simulink model "rpoco16"  (R2013a)
settings: Solver=VariableStepDiscrete  SolverMode=SingleTasking  StartTime=0.0  StopTime=10.0  RelTol=1e-3
libraries: xbsIndex_r4 x7152, casper_library_misc x156, casper_library_multipliers x68, casper_library_sources x8, xps_library x5, casper_library_delays x1
(part 3 of 84)

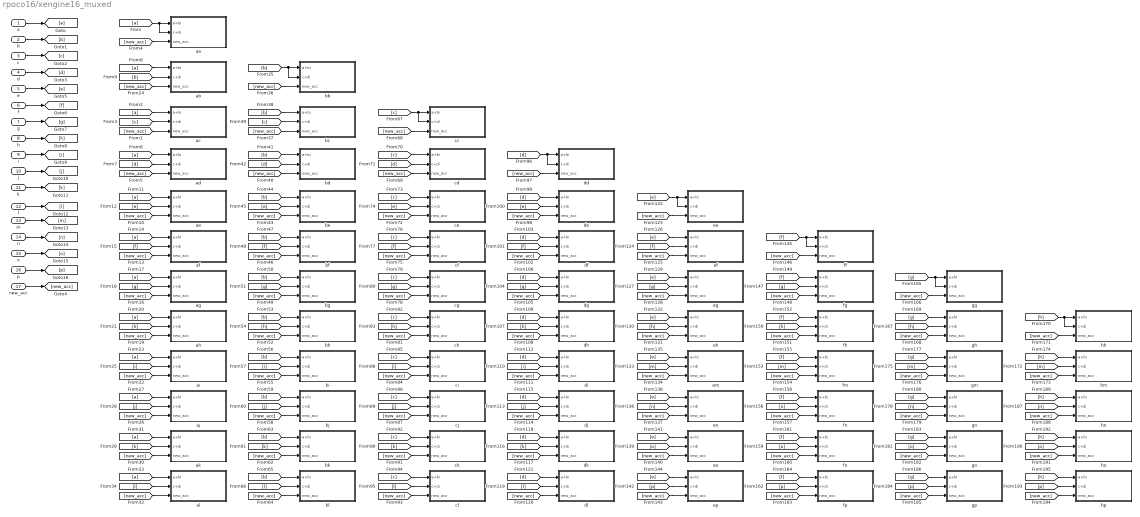
== system rpoco16/xengine16_muxed ==
  a : Inport
  b : Inport  Port=2
  c : Inport  Port=3
  d : Inport  Port=4
  e : Inport  Port=5
  f : Inport  Port=6
  g : Inport  Port=7
  h : Inport  Port=8
  i : Inport  Port=9
  j : Inport  Port=10
  k : Inport  Port=11
  l : Inport  Port=12
  m : Inport  Port=13
  n : Inport  Port=14
  o : Inport  Port=15
  p : Inport  Port=16
  new_acc : Inport  Port=17
  aa : Subsystem
  ab : Subsystem
  ac : Subsystem
  ad : Subsystem
  ae : Subsystem
  af : Subsystem
  ag : Subsystem
  ah : Subsystem
  ai : Subsystem
  aj : Subsystem
  ak : Subsystem
  al : Subsystem
  bb : Subsystem
  bc : Subsystem
  bd : Subsystem
  be : Subsystem
  bf : Subsystem
  bg : Subsystem
  bh : Subsystem
  bi : Subsystem
  bj : Subsystem
  bk : Subsystem
  bl : Subsystem
  cc : Subsystem
  cd : Subsystem
  ce : Subsystem
  cf : Subsystem
  cg : Subsystem
  ch : Subsystem
  ci : Subsystem
  cj : Subsystem
  ck : Subsystem
  cl : Subsystem
  dd : Subsystem
  de : Subsystem
  df : Subsystem
  dg : Subsystem
  dh : Subsystem
  di : Subsystem
  dj : Subsystem
  dk : Subsystem
  dl : Subsystem
  ee : Subsystem
  ef : Subsystem
  eg : Subsystem
  eh : Subsystem
  em : Subsystem
  en : Subsystem
  eo : Subsystem
  ep : Subsystem
  ff : Subsystem
  fg : Subsystem
  fh : Subsystem
  fm : Subsystem
  fn : Subsystem
  fo : Subsystem
  fp : Subsystem
  gg : Subsystem
  gh : Subsystem
  gm : Subsystem
  gn : Subsystem
  go : Subsystem
  gp : Subsystem
  hh : Subsystem
  hm : Subsystem
  hn : Subsystem
  ho : Subsystem
  hp : Subsystem
  wires:
  a/1 -> [a]
  b/1 -> [b]
  c/1 -> [c]
  d/1 -> [d]
  new_acc/1 -> [new_acc]
  [a] -> aa/2(c+di), aa/1(a+bi)
  [new_acc] -> aa/3(new_acc)
  e/1 -> [e]
  f/1 -> [f]
  g/1 -> [g]
  h/1 -> [h]
  [new_acc] -> ab/3(new_acc)
  [a] -> ab/1(a+bi)
  [b] -> ab/2(c+di)
  p/1 -> [p]
  o/1 -> [o]
  n/1 -> [n]
  m/1 -> [m]
  l/1 -> [l]
  k/1 -> [k]
  j/1 -> [j]
  i/1 -> [i]
  [new_acc] -> ac/3(new_acc)
  [a] -> ac/1(a+bi)
  [c] -> ac/2(c+di)
  [new_acc] -> ad/3(new_acc)
  [a] -> ad/1(a+bi)
  [d] -> ad/2(c+di)
  [new_acc] -> ae/3(new_acc)
  [a] -> ae/1(a+bi)
  [e] -> ae/2(c+di)
  [new_acc] -> af/3(new_acc)
  [a] -> af/1(a+bi)
  [f] -> af/2(c+di)
  [new_acc] -> ag/3(new_acc)
  [a] -> ag/1(a+bi)
  [g] -> ag/2(c+di)
  [new_acc] -> ah/3(new_acc)
  [a] -> ah/1(a+bi)
  [h] -> ah/2(c+di)
  [new_acc] -> ai/3(new_acc)
  [a] -> ai/1(a+bi)
  [i] -> ai/2(c+di)
  [new_acc] -> aj/3(new_acc)
  [a] -> aj/1(a+bi)
  [j] -> aj/2(c+di)
  [new_acc] -> al/3(new_acc)
  [a] -> al/1(a+bi)
  [l] -> al/2(c+di)
  [b] -> bb/1(a+bi), bb/2(c+di)
  [new_acc] -> bb/3(new_acc)
  [new_acc] -> bc/3(new_acc)
  [b] -> bc/1(a+bi)
  [c] -> bc/2(c+di)
  [new_acc] -> bd/3(new_acc)
  [b] -> bd/1(a+bi)
  [d] -> bd/2(c+di)
  [new_acc] -> be/3(new_acc)
  [b] -> be/1(a+bi)
  [e] -> be/2(c+di)
  [new_acc] -> bf/3(new_acc)
  [b] -> bf/1(a+bi)
  [f] -> bf/2(c+di)
  [new_acc] -> bg/3(new_acc)
  [b] -> bg/1(a+bi)
  [g] -> bg/2(c+di)
  [new_acc] -> bh/3(new_acc)
  [b] -> bh/1(a+bi)
  [h] -> bh/2(c+di)
  [new_acc] -> bi/3(new_acc)
  [b] -> bi/1(a+bi)
  [i] -> bi/2(c+di)
  [new_acc] -> bj/3(new_acc)
  [b] -> bj/1(a+bi)
  [j] -> bj/2(c+di)
  [new_acc] -> bl/3(new_acc)
  [b] -> bl/1(a+bi)
  [l] -> bl/2(c+di)
  [c] -> cc/2(c+di), cc/1(a+bi)
  [new_acc] -> cc/3(new_acc)
  [new_acc] -> cd/3(new_acc)
  [c] -> cd/1(a+bi)
  [d] -> cd/2(c+di)
  [new_acc] -> ce/3(new_acc)
  [c] -> ce/1(a+bi)
  [e] -> ce/2(c+di)
  [new_acc] -> cf/3(new_acc)
  [c] -> cf/1(a+bi)
  [f] -> cf/2(c+di)
  [new_acc] -> cg/3(new_acc)
  [c] -> cg/1(a+bi)
  [g] -> cg/2(c+di)
  [new_acc] -> ch/3(new_acc)
  [c] -> ch/1(a+bi)
  [h] -> ch/2(c+di)
  [new_acc] -> ci/3(new_acc)
  [c] -> ci/1(a+bi)
  [i] -> ci/2(c+di)
  [new_acc] -> cj/3(new_acc)
  [c] -> cj/1(a+bi)
  [j] -> cj/2(c+di)
  [new_acc] -> cl/3(new_acc)
  [c] -> cl/1(a+bi)
  [l] -> cl/2(c+di)
  [d] -> dd/1(a+bi), dd/2(c+di)
  [new_acc] -> dd/3(new_acc)
  [new_acc] -> de/3(new_acc)
  [d] -> de/1(a+bi)
  [e] -> de/2(c+di)
  [new_acc] -> df/3(new_acc)
  [d] -> df/1(a+bi)
  [f] -> df/2(c+di)
  [new_acc] -> dg/3(new_acc)
  [d] -> dg/1(a+bi)
  [g] -> dg/2(c+di)
  [new_acc] -> dh/3(new_acc)
  [d] -> dh/1(a+bi)
  [h] -> dh/2(c+di)
  [new_acc] -> di/3(new_acc)
  [d] -> di/1(a+bi)
  [i] -> di/2(c+di)
  [new_acc] -> dj/3(new_acc)
  [d] -> dj/1(a+bi)
  [j] -> dj/2(c+di)
  [new_acc] -> dl/3(new_acc)
  [d] -> dl/1(a+bi)
  [l] -> dl/2(c+di)
  [e] -> ee/2(c+di), ee/1(a+bi)
  [new_acc] -> ee/3(new_acc)
  [new_acc] -> ef/3(new_acc)
  [e] -> ef/1(a+bi)
  [f] -> ef/2(c+di)
  [new_acc] -> eg/3(new_acc)
  [e] -> eg/1(a+bi)
  [g] -> eg/2(c+di)
  [new_acc] -> eh/3(new_acc)
  [e] -> eh/1(a+bi)
  [h] -> eh/2(c+di)
  [new_acc] -> em/3(new_acc)
  [e] -> em/1(a+bi)
  [m] -> em/2(c+di)
  [new_acc] -> en/3(new_acc)
  [e] -> en/1(a+bi)
  [n] -> en/2(c+di)
  [new_acc] -> eo/3(new_acc)
  [e] -> eo/1(a+bi)
  [o] -> eo/2(c+di)
  [new_acc] -> ep/3(new_acc)
  [e] -> ep/1(a+bi)
  [p] -> ep/2(c+di)
  [f] -> ff/1(a+bi), ff/2(c+di)
  [new_acc] -> fg/3(new_acc)
  [f] -> fg/1(a+bi)
  [g] -> fg/2(c+di)
  [new_acc] -> ff/3(new_acc)
  [new_acc] -> fh/3(new_acc)
  [f] -> fh/1(a+bi)
  [h] -> fh/2(c+di)
  [new_acc] -> fm/3(new_acc)
  [f] -> fm/1(a+bi)
  [m] -> fm/2(c+di)
  [new_acc] -> fn/3(new_acc)
  [f] -> fn/1(a+bi)
  [n] -> fn/2(c+di)
  [new_acc] -> fo/3(new_acc)
  [f] -> fo/1(a+bi)
  [o] -> fo/2(c+di)
  [new_acc] -> fp/3(new_acc)
  [f] -> fp/1(a+bi)
  [p] -> fp/2(c+di)
  [g] -> gg/2(c+di), gg/1(a+bi)
  [new_acc] -> gg/3(new_acc)
  [new_acc] -> gh/3(new_acc)
  [g] -> gh/1(a+bi)
  [h] -> gh/2(c+di)
  [h] -> hh/1(a+bi), hh/2(c+di)
  [new_acc] -> hh/3(new_acc)
  [new_acc] -> hm/3(new_acc)
  [h] -> hm/1(a+bi)
  [m] -> hm/2(c+di)
  [new_acc] -> gm/3(new_acc)
  [g] -> gm/1(a+bi)
  [m] -> gm/2(c+di)
  [new_acc] -> gn/3(new_acc)
  [g] -> gn/1(a+bi)
  [n] -> gn/2(c+di)
  [new_acc] -> go/3(new_acc)
  [g] -> go/1(a+bi)
  [o] -> go/2(c+di)
  [new_acc] -> gp/3(new_acc)
  [g] -> gp/1(a+bi)
  [p] -> gp/2(c+di)
  [new_acc] -> hn/3(new_acc)
  [h] -> hn/1(a+bi)
  [n] -> hn/2(c+di)
  [new_acc] -> ho/3(new_acc)
  [h] -> ho/1(a+bi)
  [o] -> ho/2(c+di)
  [new_acc] -> hp/3(new_acc)
  [h] -> hp/1(a+bi)
  [p] -> hp/2(c+di)
  [new_acc] -> ak/3(new_acc)
  [a] -> ak/1(a+bi)
  [k] -> ak/2(c+di)
  [new_acc] -> bk/3(new_acc)
  [b] -> bk/1(a+bi)
  [k] -> bk/2(c+di)
  [new_acc] -> ck/3(new_acc)
  [c] -> ck/1(a+bi)
  [k] -> ck/2(c+di)
  [new_acc] -> dk/3(new_acc)
  [d] -> dk/1(a+bi)
  [k] -> dk/2(c+di)

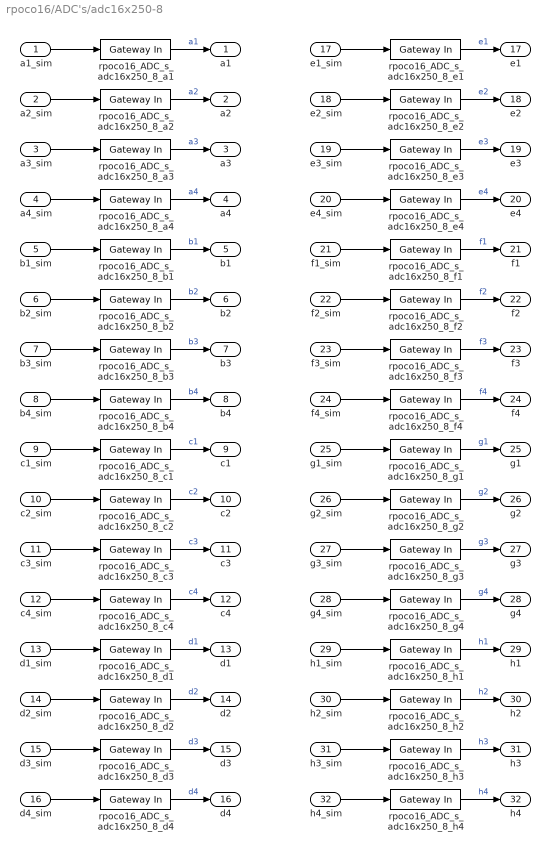
== system rpoco16/ADC's/adc16x250-8 ==
  a1_sim : Inport
  a2_sim : Inport  Port=2
  a3_sim : Inport  Port=3
  a4_sim : Inport  Port=4
  b1_sim : Inport  Port=5
  b2_sim : Inport  Port=6
  b3_sim : Inport  Port=7
  b4_sim : Inport  Port=8
  c1_sim : Inport  Port=9
  c2_sim : Inport  Port=10
  c3_sim : Inport  Port=11
  c4_sim : Inport  Port=12
  d1_sim : Inport  Port=13
  d2_sim : Inport  Port=14
  d3_sim : Inport  Port=15
  d4_sim : Inport  Port=16
  e1_sim : Inport  Port=17
  e2_sim : Inport  Port=18
  e3_sim : Inport  Port=19
  e4_sim : Inport  Port=20
  f1_sim : Inport  Port=21
  f2_sim : Inport  Port=22
  f3_sim : Inport  Port=23
  f4_sim : Inport  Port=24
  g1_sim : Inport  Port=25
  g2_sim : Inport  Port=26
  g3_sim : Inport  Port=27
  g4_sim : Inport  Port=28
  h1_sim : Inport  Port=29
  h2_sim : Inport  Port=30
  h3_sim : Inport  Port=31
  h4_sim : Inport  Port=32
  rpoco16_ADC_s_adc16x250_8_a{1..4} (4 alike) : xbsIndex_r4/Gateway In  gui_display_data_type=Fixed-point  arith_type="Signed  (2's comp)"  n_bits=8  bin_pt=7  preci_type=Single  exp_width=8  frac_width=24  quantization="Round  (unbiased: +/- Inf)"  overflow=Saturate  period=1  dbl_ovrd=off  timing_constraint=None  locs_specified=off  LOCs={}  UseAsADC=off  ADCChannel='1'  inherit_from_input=off  hdl_port=on  block_type=gatewayin
  rpoco16_ADC_s_adc16x250_8_b{1..4} (4 alike) : xbsIndex_r4/Gateway In  gui_display_data_type=Fixed-point  arith_type="Signed  (2's comp)"  n_bits=8  bin_pt=7  preci_type=Single  exp_width=8  frac_width=24  quantization="Round  (unbiased: +/- Inf)"  overflow=Saturate  period=1  dbl_ovrd=off  timing_constraint=None  locs_specified=off  LOCs={}  UseAsADC=off  ADCChannel='1'  inherit_from_input=off  hdl_port=on  block_type=gatewayin
  rpoco16_ADC_s_adc16x250_8_c{1..4} (4 alike) : xbsIndex_r4/Gateway In  gui_display_data_type=Fixed-point  arith_type="Signed  (2's comp)"  n_bits=8  bin_pt=7  preci_type=Single  exp_width=8  frac_width=24  quantization="Round  (unbiased: +/- Inf)"  overflow=Saturate  period=1  dbl_ovrd=off  timing_constraint=None  locs_specified=off  LOCs={}  UseAsADC=off  ADCChannel='1'  inherit_from_input=off  hdl_port=on  block_type=gatewayin
  rpoco16_ADC_s_adc16x250_8_d{1..4} (4 alike) : xbsIndex_r4/Gateway In  gui_display_data_type=Fixed-point  arith_type="Signed  (2's comp)"  n_bits=8  bin_pt=7  preci_type=Single  exp_width=8  frac_width=24  quantization="Round  (unbiased: +/- Inf)"  overflow=Saturate  period=1  dbl_ovrd=off  timing_constraint=None  locs_specified=off  LOCs={}  UseAsADC=off  ADCChannel='1'  inherit_from_input=off  hdl_port=on  block_type=gatewayin
  rpoco16_ADC_s_adc16x250_8_e{1..4} (4 alike) : xbsIndex_r4/Gateway In  gui_display_data_type=Fixed-point  arith_type="Signed  (2's comp)"  n_bits=8  bin_pt=7  preci_type=Single  exp_width=8  frac_width=24  quantization="Round  (unbiased: +/- Inf)"  overflow=Saturate  period=1  dbl_ovrd=off  timing_constraint=None  locs_specified=off  LOCs={}  UseAsADC=off  ADCChannel='1'  inherit_from_input=off  hdl_port=on  block_type=gatewayin
  rpoco16_ADC_s_adc16x250_8_f{1..4} (4 alike) : xbsIndex_r4/Gateway In  gui_display_data_type=Fixed-point  arith_type="Signed  (2's comp)"  n_bits=8  bin_pt=7  preci_type=Single  exp_width=8  frac_width=24  quantization="Round  (unbiased: +/- Inf)"  overflow=Saturate  period=1  dbl_ovrd=off  timing_constraint=None  locs_specified=off  LOCs={}  UseAsADC=off  ADCChannel='1'  inherit_from_input=off  hdl_port=on  block_type=gatewayin
  rpoco16_ADC_s_adc16x250_8_g{1..4} (4 alike) : xbsIndex_r4/Gateway In  gui_display_data_type=Fixed-point  arith_type="Signed  (2's comp)"  n_bits=8  bin_pt=7  preci_type=Single  exp_width=8  frac_width=24  quantization="Round  (unbiased: +/- Inf)"  overflow=Saturate  period=1  dbl_ovrd=off  timing_constraint=None  locs_specified=off  LOCs={}  UseAsADC=off  ADCChannel='1'  inherit_from_input=off  hdl_port=on  block_type=gatewayin
  rpoco16_ADC_s_adc16x250_8_h{1..4} (4 alike) : xbsIndex_r4/Gateway In  gui_display_data_type=Fixed-point  arith_type="Signed  (2's comp)"  n_bits=8  bin_pt=7  preci_type=Single  exp_width=8  frac_width=24  quantization="Round  (unbiased: +/- Inf)"  overflow=Saturate  period=1  dbl_ovrd=off  timing_constraint=None  locs_specified=off  LOCs={}  UseAsADC=off  ADCChannel='1'  inherit_from_input=off  hdl_port=on  block_type=gatewayin
  a1 : Outport
  a2 : Outport  Port=2
  a3 : Outport  Port=3
  a4 : Outport  Port=4
  b1 : Outport  Port=5
  b2 : Outport  Port=6
  b3 : Outport  Port=7
  b4 : Outport  Port=8
  c1 : Outport  Port=9
  c2 : Outport  Port=10
  c3 : Outport  Port=11
  c4 : Outport  Port=12
  d1 : Outport  Port=13
  d2 : Outport  Port=14
  d3 : Outport  Port=15
  d4 : Outport  Port=16
  e1 : Outport  Port=17
  e2 : Outport  Port=18
  e3 : Outport  Port=19
  e4 : Outport  Port=20
  f1 : Outport  Port=21
  f2 : Outport  Port=22
  f3 : Outport  Port=23
  f4 : Outport  Port=24
  g1 : Outport  Port=25
  g2 : Outport  Port=26
  g3 : Outport  Port=27
  g4 : Outport  Port=28
  h1 : Outport  Port=29
  h2 : Outport  Port=30
  h3 : Outport  Port=31
  h4 : Outport  Port=32
  wires:
  a1_sim/1 -> rpoco16_ADC_s_adc16x250_8_a1/1
  rpoco16_ADC_s_adc16x250_8_a1/1 -> a1/1  "a1"
  a2_sim/1 -> rpoco16_ADC_s_adc16x250_8_a2/1
  rpoco16_ADC_s_adc16x250_8_a2/1 -> a2/1  "a2"
  a3_sim/1 -> rpoco16_ADC_s_adc16x250_8_a3/1
  rpoco16_ADC_s_adc16x250_8_a3/1 -> a3/1  "a3"
  a4_sim/1 -> rpoco16_ADC_s_adc16x250_8_a4/1
  rpoco16_ADC_s_adc16x250_8_a4/1 -> a4/1  "a4"
  b1_sim/1 -> rpoco16_ADC_s_adc16x250_8_b1/1
  rpoco16_ADC_s_adc16x250_8_b1/1 -> b1/1  "b1"
  b2_sim/1 -> rpoco16_ADC_s_adc16x250_8_b2/1
  rpoco16_ADC_s_adc16x250_8_b2/1 -> b2/1  "b2"
  b3_sim/1 -> rpoco16_ADC_s_adc16x250_8_b3/1
  rpoco16_ADC_s_adc16x250_8_b3/1 -> b3/1  "b3"
  b4_sim/1 -> rpoco16_ADC_s_adc16x250_8_b4/1
  rpoco16_ADC_s_adc16x250_8_b4/1 -> b4/1  "b4"
  c1_sim/1 -> rpoco16_ADC_s_adc16x250_8_c1/1
  rpoco16_ADC_s_adc16x250_8_c1/1 -> c1/1  "c1"
  c2_sim/1 -> rpoco16_ADC_s_adc16x250_8_c2/1
  rpoco16_ADC_s_adc16x250_8_c2/1 -> c2/1  "c2"
  c3_sim/1 -> rpoco16_ADC_s_adc16x250_8_c3/1
  rpoco16_ADC_s_adc16x250_8_c3/1 -> c3/1  "c3"
  c4_sim/1 -> rpoco16_ADC_s_adc16x250_8_c4/1
  rpoco16_ADC_s_adc16x250_8_c4/1 -> c4/1  "c4"
  d1_sim/1 -> rpoco16_ADC_s_adc16x250_8_d1/1
  rpoco16_ADC_s_adc16x250_8_d1/1 -> d1/1  "d1"
  d2_sim/1 -> rpoco16_ADC_s_adc16x250_8_d2/1
  rpoco16_ADC_s_adc16x250_8_d2/1 -> d2/1  "d2"
  d3_sim/1 -> rpoco16_ADC_s_adc16x250_8_d3/1
  rpoco16_ADC_s_adc16x250_8_d3/1 -> d3/1  "d3"
  d4_sim/1 -> rpoco16_ADC_s_adc16x250_8_d4/1
  rpoco16_ADC_s_adc16x250_8_d4/1 -> d4/1  "d4"
  e1_sim/1 -> rpoco16_ADC_s_adc16x250_8_e1/1
  rpoco16_ADC_s_adc16x250_8_e1/1 -> e1/1  "e1"
  e2_sim/1 -> rpoco16_ADC_s_adc16x250_8_e2/1
  rpoco16_ADC_s_adc16x250_8_e2/1 -> e2/1  "e2"
  e3_sim/1 -> rpoco16_ADC_s_adc16x250_8_e3/1
  rpoco16_ADC_s_adc16x250_8_e3/1 -> e3/1  "e3"
  e4_sim/1 -> rpoco16_ADC_s_adc16x250_8_e4/1
  rpoco16_ADC_s_adc16x250_8_e4/1 -> e4/1  "e4"
  f1_sim/1 -> rpoco16_ADC_s_adc16x250_8_f1/1
  rpoco16_ADC_s_adc16x250_8_f1/1 -> f1/1  "f1"
  f2_sim/1 -> rpoco16_ADC_s_adc16x250_8_f2/1
  rpoco16_ADC_s_adc16x250_8_f2/1 -> f2/1  "f2"
  f3_sim/1 -> rpoco16_ADC_s_adc16x250_8_f3/1
  rpoco16_ADC_s_adc16x250_8_f3/1 -> f3/1  "f3"
  f4_sim/1 -> rpoco16_ADC_s_adc16x250_8_f4/1
  rpoco16_ADC_s_adc16x250_8_f4/1 -> f4/1  "f4"
  g1_sim/1 -> rpoco16_ADC_s_adc16x250_8_g1/1
  rpoco16_ADC_s_adc16x250_8_g1/1 -> g1/1  "g1"
  g2_sim/1 -> rpoco16_ADC_s_adc16x250_8_g2/1
  rpoco16_ADC_s_adc16x250_8_g2/1 -> g2/1  "g2"
  g3_sim/1 -> rpoco16_ADC_s_adc16x250_8_g3/1
  rpoco16_ADC_s_adc16x250_8_g3/1 -> g3/1  "g3"
  g4_sim/1 -> rpoco16_ADC_s_adc16x250_8_g4/1
  rpoco16_ADC_s_adc16x250_8_g4/1 -> g4/1  "g4"
  h1_sim/1 -> rpoco16_ADC_s_adc16x250_8_h1/1
  rpoco16_ADC_s_adc16x250_8_h1/1 -> h1/1  "h1"
  h2_sim/1 -> rpoco16_ADC_s_adc16x250_8_h2/1
  rpoco16_ADC_s_adc16x250_8_h2/1 -> h2/1  "h2"
  h3_sim/1 -> rpoco16_ADC_s_adc16x250_8_h3/1
  rpoco16_ADC_s_adc16x250_8_h3/1 -> h3/1  "h3"
  h4_sim/1 -> rpoco16_ADC_s_adc16x250_8_h4/1
  rpoco16_ADC_s_adc16x250_8_h4/1 -> h4/1  "h4"

== system rpoco16/ADC's/sat ==
  In2 : Inport
  Constant3 : xbsIndex_r4/Constant  const=-1  gui_display_data_type=Fixed-point  arith_type=Signed (2's comp)  n_bits=8  bin_pt=7  preci_type=Single  exp_width=8  frac_width=24  explicit_period=off  period=1  equ=P=C  opselect=C  inp2=PCIN>>17  opr=+  inp1=P  carry=CIN  dbl_ovrd=off  block_type=constant
      settings: block_version=11.4
  Constant4 : xbsIndex_r4/Constant  const=-127/128.  gui_display_data_type=Fixed-point  arith_type=Signed (2's comp)  n_bits=8  bin_pt=7  preci_type=Single  exp_width=8  frac_width=24  explicit_period=off  period=1  equ=P=C  opselect=C  inp2=PCIN>>17  opr=+  inp1=P  carry=CIN  dbl_ovrd=off  block_type=constant
      settings: block_version=11.4
  Mux1 : xbsIndex_r4/Mux  inputs=2  en=off  latency=0  precision=Full  arith_type=Unsigned  n_bits=16  bin_pt=14  quantization=Truncate  overflow=Wrap  dbl_ovrd=off  block_type=mux
      settings: block_version=11.4
  Relational : xbsIndex_r4/Relational  mode=a=b  en=off  latency=0  dbl_ovrd=off  block_type=relational
  Out1 : Outport
  wires:
  Constant3/1 -> Relational/1
  Relational/1 -> Mux1/1
  Constant4/1 -> Mux1/3
  Mux1/1 -> Out1/1
  In2/1 -> [d]
  [d] -> Relational/2
  [d] -> Mux1/2

== system rpoco16/ADC's/sat1 ==
  In2 : Inport
  Constant3 : xbsIndex_r4/Constant  const=-1  gui_display_data_type=Fixed-point  arith_type=Signed (2's comp)  n_bits=8  bin_pt=7  preci_type=Single  exp_width=8  frac_width=24  explicit_period=off  period=1  equ=P=C  opselect=C  inp2=PCIN>>17  opr=+  inp1=P  carry=CIN  dbl_ovrd=off  block_type=constant
      settings: block_version=11.4
  Constant4 : xbsIndex_r4/Constant  const=-127/128.  gui_display_data_type=Fixed-point  arith_type=Signed (2's comp)  n_bits=8  bin_pt=7  preci_type=Single  exp_width=8  frac_width=24  explicit_period=off  period=1  equ=P=C  opselect=C  inp2=PCIN>>17  opr=+  inp1=P  carry=CIN  dbl_ovrd=off  block_type=constant
      settings: block_version=11.4
  Mux1 : xbsIndex_r4/Mux  inputs=2  en=off  latency=0  precision=Full  arith_type=Unsigned  n_bits=16  bin_pt=14  quantization=Truncate  overflow=Wrap  dbl_ovrd=off  block_type=mux
      settings: block_version=11.4
  Relational : xbsIndex_r4/Relational  mode=a=b  en=off  latency=0  dbl_ovrd=off  block_type=relational
  Out1 : Outport
  wires:
  [d] -> Mux1/2
  [d] -> Relational/2
  In2/1 -> [d]
  Mux1/1 -> Out1/1
  Constant4/1 -> Mux1/3
  Relational/1 -> Mux1/1
  Constant3/1 -> Relational/1

== system rpoco16/ADC's/sat10 ==
  In2 : Inport
  Constant3 : xbsIndex_r4/Constant  const=-1  gui_display_data_type=Fixed-point  arith_type=Signed (2's comp)  n_bits=8  bin_pt=7  preci_type=Single  exp_width=8  frac_width=24  explicit_period=off  period=1  equ=P=C  opselect=C  inp2=PCIN>>17  opr=+  inp1=P  carry=CIN  dbl_ovrd=off  block_type=constant
      settings: block_version=11.4
  Constant4 : xbsIndex_r4/Constant  const=-127/128.  gui_display_data_type=Fixed-point  arith_type=Signed (2's comp)  n_bits=8  bin_pt=7  preci_type=Single  exp_width=8  frac_width=24  explicit_period=off  period=1  equ=P=C  opselect=C  inp2=PCIN>>17  opr=+  inp1=P  carry=CIN  dbl_ovrd=off  block_type=constant
      settings: block_version=11.4
  Mux1 : xbsIndex_r4/Mux  inputs=2  en=off  latency=0  precision=Full  arith_type=Unsigned  n_bits=16  bin_pt=14  quantization=Truncate  overflow=Wrap  dbl_ovrd=off  block_type=mux
      settings: block_version=11.4
  Relational : xbsIndex_r4/Relational  mode=a=b  en=off  latency=0  dbl_ovrd=off  block_type=relational
  Out1 : Outport
  wires:
  Constant3/1 -> Relational/1
  Relational/1 -> Mux1/1
  Constant4/1 -> Mux1/3
  Mux1/1 -> Out1/1
  In2/1 -> [d]
  [d] -> Relational/2
  [d] -> Mux1/2

== system rpoco16/ADC's/sat11 ==
  In2 : Inport
  Constant3 : xbsIndex_r4/Constant  const=-1  gui_display_data_type=Fixed-point  arith_type=Signed (2's comp)  n_bits=8  bin_pt=7  preci_type=Single  exp_width=8  frac_width=24  explicit_period=off  period=1  equ=P=C  opselect=C  inp2=PCIN>>17  opr=+  inp1=P  carry=CIN  dbl_ovrd=off  block_type=constant
      settings: block_version=11.4
  Constant4 : xbsIndex_r4/Constant  const=-127/128.  gui_display_data_type=Fixed-point  arith_type=Signed (2's comp)  n_bits=8  bin_pt=7  preci_type=Single  exp_width=8  frac_width=24  explicit_period=off  period=1  equ=P=C  opselect=C  inp2=PCIN>>17  opr=+  inp1=P  carry=CIN  dbl_ovrd=off  block_type=constant
      settings: block_version=11.4
  Mux1 : xbsIndex_r4/Mux  inputs=2  en=off  latency=0  precision=Full  arith_type=Unsigned  n_bits=16  bin_pt=14  quantization=Truncate  overflow=Wrap  dbl_ovrd=off  block_type=mux
      settings: block_version=11.4
  Relational : xbsIndex_r4/Relational  mode=a=b  en=off  latency=0  dbl_ovrd=off  block_type=relational
  Out1 : Outport
  wires:
  [d] -> Mux1/2
  [d] -> Relational/2
  In2/1 -> [d]
  Mux1/1 -> Out1/1
  Constant4/1 -> Mux1/3
  Relational/1 -> Mux1/1
  Constant3/1 -> Relational/1

== system rpoco16/ADC's/sat12 ==
  In2 : Inport
  Constant3 : xbsIndex_r4/Constant  const=-1  gui_display_data_type=Fixed-point  arith_type=Signed (2's comp)  n_bits=8  bin_pt=7  preci_type=Single  exp_width=8  frac_width=24  explicit_period=off  period=1  equ=P=C  opselect=C  inp2=PCIN>>17  opr=+  inp1=P  carry=CIN  dbl_ovrd=off  block_type=constant
      settings: block_version=11.4
  Constant4 : xbsIndex_r4/Constant  const=-127/128.  gui_display_data_type=Fixed-point  arith_type=Signed (2's comp)  n_bits=8  bin_pt=7  preci_type=Single  exp_width=8  frac_width=24  explicit_period=off  period=1  equ=P=C  opselect=C  inp2=PCIN>>17  opr=+  inp1=P  carry=CIN  dbl_ovrd=off  block_type=constant
      settings: block_version=11.4
  Mux1 : xbsIndex_r4/Mux  inputs=2  en=off  latency=0  precision=Full  arith_type=Unsigned  n_bits=16  bin_pt=14  quantization=Truncate  overflow=Wrap  dbl_ovrd=off  block_type=mux
      settings: block_version=11.4
  Relational : xbsIndex_r4/Relational  mode=a=b  en=off  latency=0  dbl_ovrd=off  block_type=relational
  Out1 : Outport
  wires:
  Constant3/1 -> Relational/1
  Relational/1 -> Mux1/1
  Constant4/1 -> Mux1/3
  Mux1/1 -> Out1/1
  In2/1 -> [d]
  [d] -> Relational/2
  [d] -> Mux1/2

== system rpoco16/ADC's/sat13 ==
  In2 : Inport
  Constant3 : xbsIndex_r4/Constant  const=-1  gui_display_data_type=Fixed-point  arith_type=Signed (2's comp)  n_bits=8  bin_pt=7  preci_type=Single  exp_width=8  frac_width=24  explicit_period=off  period=1  equ=P=C  opselect=C  inp2=PCIN>>17  opr=+  inp1=P  carry=CIN  dbl_ovrd=off  block_type=constant
      settings: block_version=11.4
  Constant4 : xbsIndex_r4/Constant  const=-127/128.  gui_display_data_type=Fixed-point  arith_type=Signed (2's comp)  n_bits=8  bin_pt=7  preci_type=Single  exp_width=8  frac_width=24  explicit_period=off  period=1  equ=P=C  opselect=C  inp2=PCIN>>17  opr=+  inp1=P  carry=CIN  dbl_ovrd=off  block_type=constant
      settings: block_version=11.4
  Mux1 : xbsIndex_r4/Mux  inputs=2  en=off  latency=0  precision=Full  arith_type=Unsigned  n_bits=16  bin_pt=14  quantization=Truncate  overflow=Wrap  dbl_ovrd=off  block_type=mux
      settings: block_version=11.4
  Relational : xbsIndex_r4/Relational  mode=a=b  en=off  latency=0  dbl_ovrd=off  block_type=relational
  Out1 : Outport
  wires:
  [d] -> Mux1/2
  [d] -> Relational/2
  In2/1 -> [d]
  Mux1/1 -> Out1/1
  Constant4/1 -> Mux1/3
  Relational/1 -> Mux1/1
  Constant3/1 -> Relational/1

== system rpoco16/ADC's/sat14 ==
  In2 : Inport
  Constant3 : xbsIndex_r4/Constant  const=-1  gui_display_data_type=Fixed-point  arith_type=Signed (2's comp)  n_bits=8  bin_pt=7  preci_type=Single  exp_width=8  frac_width=24  explicit_period=off  period=1  equ=P=C  opselect=C  inp2=PCIN>>17  opr=+  inp1=P  carry=CIN  dbl_ovrd=off  block_type=constant
      settings: block_version=11.4
  Constant4 : xbsIndex_r4/Constant  const=-127/128.  gui_display_data_type=Fixed-point  arith_type=Signed (2's comp)  n_bits=8  bin_pt=7  preci_type=Single  exp_width=8  frac_width=24  explicit_period=off  period=1  equ=P=C  opselect=C  inp2=PCIN>>17  opr=+  inp1=P  carry=CIN  dbl_ovrd=off  block_type=constant
      settings: block_version=11.4
  Mux1 : xbsIndex_r4/Mux  inputs=2  en=off  latency=0  precision=Full  arith_type=Unsigned  n_bits=16  bin_pt=14  quantization=Truncate  overflow=Wrap  dbl_ovrd=off  block_type=mux
      settings: block_version=11.4
  Relational : xbsIndex_r4/Relational  mode=a=b  en=off  latency=0  dbl_ovrd=off  block_type=relational
  Out1 : Outport
  wires:
  Constant3/1 -> Relational/1
  Relational/1 -> Mux1/1
  Constant4/1 -> Mux1/3
  Mux1/1 -> Out1/1
  In2/1 -> [d]
  [d] -> Relational/2
  [d] -> Mux1/2

== system rpoco16/ADC's/sat15 ==
  In2 : Inport
  Constant3 : xbsIndex_r4/Constant  const=-1  gui_display_data_type=Fixed-point  arith_type=Signed (2's comp)  n_bits=8  bin_pt=7  preci_type=Single  exp_width=8  frac_width=24  explicit_period=off  period=1  equ=P=C  opselect=C  inp2=PCIN>>17  opr=+  inp1=P  carry=CIN  dbl_ovrd=off  block_type=constant
      settings: block_version=11.4
  Constant4 : xbsIndex_r4/Constant  const=-127/128.  gui_display_data_type=Fixed-point  arith_type=Signed (2's comp)  n_bits=8  bin_pt=7  preci_type=Single  exp_width=8  frac_width=24  explicit_period=off  period=1  equ=P=C  opselect=C  inp2=PCIN>>17  opr=+  inp1=P  carry=CIN  dbl_ovrd=off  block_type=constant
      settings: block_version=11.4
  Mux1 : xbsIndex_r4/Mux  inputs=2  en=off  latency=0  precision=Full  arith_type=Unsigned  n_bits=16  bin_pt=14  quantization=Truncate  overflow=Wrap  dbl_ovrd=off  block_type=mux
      settings: block_version=11.4
  Relational : xbsIndex_r4/Relational  mode=a=b  en=off  latency=0  dbl_ovrd=off  block_type=relational
  Out1 : Outport
  wires:
  [d] -> Mux1/2
  [d] -> Relational/2
  In2/1 -> [d]
  Mux1/1 -> Out1/1
  Constant4/1 -> Mux1/3
  Relational/1 -> Mux1/1
  Constant3/1 -> Relational/1

== system rpoco16/ADC's/sat2 ==
  In2 : Inport
  Constant3 : xbsIndex_r4/Constant  const=-1  gui_display_data_type=Fixed-point  arith_type=Signed (2's comp)  n_bits=8  bin_pt=7  preci_type=Single  exp_width=8  frac_width=24  explicit_period=off  period=1  equ=P=C  opselect=C  inp2=PCIN>>17  opr=+  inp1=P  carry=CIN  dbl_ovrd=off  block_type=constant
      settings: block_version=11.4
  Constant4 : xbsIndex_r4/Constant  const=-127/128.  gui_display_data_type=Fixed-point  arith_type=Signed (2's comp)  n_bits=8  bin_pt=7  preci_type=Single  exp_width=8  frac_width=24  explicit_period=off  period=1  equ=P=C  opselect=C  inp2=PCIN>>17  opr=+  inp1=P  carry=CIN  dbl_ovrd=off  block_type=constant
      settings: block_version=11.4
  Mux1 : xbsIndex_r4/Mux  inputs=2  en=off  latency=0  precision=Full  arith_type=Unsigned  n_bits=16  bin_pt=14  quantization=Truncate  overflow=Wrap  dbl_ovrd=off  block_type=mux
      settings: block_version=11.4
  Relational : xbsIndex_r4/Relational  mode=a=b  en=off  latency=0  dbl_ovrd=off  block_type=relational
  Out1 : Outport
  wires:
  Constant3/1 -> Relational/1
  Relational/1 -> Mux1/1
  Constant4/1 -> Mux1/3
  Mux1/1 -> Out1/1
  In2/1 -> [d]
  [d] -> Relational/2
  [d] -> Mux1/2

== system rpoco16/ADC's/sat3 ==
  In2 : Inport
  Constant3 : xbsIndex_r4/Constant  const=-1  gui_display_data_type=Fixed-point  arith_type=Signed (2's comp)  n_bits=8  bin_pt=7  preci_type=Single  exp_width=8  frac_width=24  explicit_period=off  period=1  equ=P=C  opselect=C  inp2=PCIN>>17  opr=+  inp1=P  carry=CIN  dbl_ovrd=off  block_type=constant
      settings: block_version=11.4
  Constant4 : xbsIndex_r4/Constant  const=-127/128.  gui_display_data_type=Fixed-point  arith_type=Signed (2's comp)  n_bits=8  bin_pt=7  preci_type=Single  exp_width=8  frac_width=24  explicit_period=off  period=1  equ=P=C  opselect=C  inp2=PCIN>>17  opr=+  inp1=P  carry=CIN  dbl_ovrd=off  block_type=constant
      settings: block_version=11.4
  Mux1 : xbsIndex_r4/Mux  inputs=2  en=off  latency=0  precision=Full  arith_type=Unsigned  n_bits=16  bin_pt=14  quantization=Truncate  overflow=Wrap  dbl_ovrd=off  block_type=mux
      settings: block_version=11.4
  Relational : xbsIndex_r4/Relational  mode=a=b  en=off  latency=0  dbl_ovrd=off  block_type=relational
  Out1 : Outport
  wires:
  [d] -> Mux1/2
  [d] -> Relational/2
  In2/1 -> [d]
  Mux1/1 -> Out1/1
  Constant4/1 -> Mux1/3
  Relational/1 -> Mux1/1
  Constant3/1 -> Relational/1

== system rpoco16/ADC's/sat4 ==
  In2 : Inport
  Constant3 : xbsIndex_r4/Constant  const=-1  gui_display_data_type=Fixed-point  arith_type=Signed (2's comp)  n_bits=8  bin_pt=7  preci_type=Single  exp_width=8  frac_width=24  explicit_period=off  period=1  equ=P=C  opselect=C  inp2=PCIN>>17  opr=+  inp1=P  carry=CIN  dbl_ovrd=off  block_type=constant
      settings: block_version=11.4
  Constant4 : xbsIndex_r4/Constant  const=-127/128.  gui_display_data_type=Fixed-point  arith_type=Signed (2's comp)  n_bits=8  bin_pt=7  preci_type=Single  exp_width=8  frac_width=24  explicit_period=off  period=1  equ=P=C  opselect=C  inp2=PCIN>>17  opr=+  inp1=P  carry=CIN  dbl_ovrd=off  block_type=constant
      settings: block_version=11.4
  Mux1 : xbsIndex_r4/Mux  inputs=2  en=off  latency=0  precision=Full  arith_type=Unsigned  n_bits=16  bin_pt=14  quantization=Truncate  overflow=Wrap  dbl_ovrd=off  block_type=mux
      settings: block_version=11.4
  Relational : xbsIndex_r4/Relational  mode=a=b  en=off  latency=0  dbl_ovrd=off  block_type=relational
  Out1 : Outport
  wires:
  Constant3/1 -> Relational/1
  Relational/1 -> Mux1/1
  Constant4/1 -> Mux1/3
  Mux1/1 -> Out1/1
  In2/1 -> [d]
  [d] -> Relational/2
  [d] -> Mux1/2

== system rpoco16/ADC's/sat5 ==
  In2 : Inport
  Constant3 : xbsIndex_r4/Constant  const=-1  gui_display_data_type=Fixed-point  arith_type=Signed (2's comp)  n_bits=8  bin_pt=7  preci_type=Single  exp_width=8  frac_width=24  explicit_period=off  period=1  equ=P=C  opselect=C  inp2=PCIN>>17  opr=+  inp1=P  carry=CIN  dbl_ovrd=off  block_type=constant
      settings: block_version=11.4
  Constant4 : xbsIndex_r4/Constant  const=-127/128.  gui_display_data_type=Fixed-point  arith_type=Signed (2's comp)  n_bits=8  bin_pt=7  preci_type=Single  exp_width=8  frac_width=24  explicit_period=off  period=1  equ=P=C  opselect=C  inp2=PCIN>>17  opr=+  inp1=P  carry=CIN  dbl_ovrd=off  block_type=constant
      settings: block_version=11.4
  Mux1 : xbsIndex_r4/Mux  inputs=2  en=off  latency=0  precision=Full  arith_type=Unsigned  n_bits=16  bin_pt=14  quantization=Truncate  overflow=Wrap  dbl_ovrd=off  block_type=mux
      settings: block_version=11.4
  Relational : xbsIndex_r4/Relational  mode=a=b  en=off  latency=0  dbl_ovrd=off  block_type=relational
  Out1 : Outport
  wires:
  [d] -> Mux1/2
  [d] -> Relational/2
  In2/1 -> [d]
  Mux1/1 -> Out1/1
  Constant4/1 -> Mux1/3
  Relational/1 -> Mux1/1
  Constant3/1 -> Relational/1

== system rpoco16/ADC's/sat6 ==
  In2 : Inport
  Constant3 : xbsIndex_r4/Constant  const=-1  gui_display_data_type=Fixed-point  arith_type=Signed (2's comp)  n_bits=8  bin_pt=7  preci_type=Single  exp_width=8  frac_width=24  explicit_period=off  period=1  equ=P=C  opselect=C  inp2=PCIN>>17  opr=+  inp1=P  carry=CIN  dbl_ovrd=off  block_type=constant
      settings: block_version=11.4
  Constant4 : xbsIndex_r4/Constant  const=-127/128.  gui_display_data_type=Fixed-point  arith_type=Signed (2's comp)  n_bits=8  bin_pt=7  preci_type=Single  exp_width=8  frac_width=24  explicit_period=off  period=1  equ=P=C  opselect=C  inp2=PCIN>>17  opr=+  inp1=P  carry=CIN  dbl_ovrd=off  block_type=constant
      settings: block_version=11.4
  Mux1 : xbsIndex_r4/Mux  inputs=2  en=off  latency=0  precision=Full  arith_type=Unsigned  n_bits=16  bin_pt=14  quantization=Truncate  overflow=Wrap  dbl_ovrd=off  block_type=mux
      settings: block_version=11.4
  Relational : xbsIndex_r4/Relational  mode=a=b  en=off  latency=0  dbl_ovrd=off  block_type=relational
  Out1 : Outport
  wires:
  Constant3/1 -> Relational/1
  Relational/1 -> Mux1/1
  Constant4/1 -> Mux1/3
  Mux1/1 -> Out1/1
  In2/1 -> [d]
  [d] -> Relational/2
  [d] -> Mux1/2

== system rpoco16/ADC's/sat7 ==
  In2 : Inport
  Constant3 : xbsIndex_r4/Constant  const=-1  gui_display_data_type=Fixed-point  arith_type=Signed (2's comp)  n_bits=8  bin_pt=7  preci_type=Single  exp_width=8  frac_width=24  explicit_period=off  period=1  equ=P=C  opselect=C  inp2=PCIN>>17  opr=+  inp1=P  carry=CIN  dbl_ovrd=off  block_type=constant
      settings: block_version=11.4
  Constant4 : xbsIndex_r4/Constant  const=-127/128.  gui_display_data_type=Fixed-point  arith_type=Signed (2's comp)  n_bits=8  bin_pt=7  preci_type=Single  exp_width=8  frac_width=24  explicit_period=off  period=1  equ=P=C  opselect=C  inp2=PCIN>>17  opr=+  inp1=P  carry=CIN  dbl_ovrd=off  block_type=constant
      settings: block_version=11.4
  Mux1 : xbsIndex_r4/Mux  inputs=2  en=off  latency=0  precision=Full  arith_type=Unsigned  n_bits=16  bin_pt=14  quantization=Truncate  overflow=Wrap  dbl_ovrd=off  block_type=mux
      settings: block_version=11.4
  Relational : xbsIndex_r4/Relational  mode=a=b  en=off  latency=0  dbl_ovrd=off  block_type=relational
  Out1 : Outport
  wires:
  [d] -> Mux1/2
  [d] -> Relational/2
  In2/1 -> [d]
  Mux1/1 -> Out1/1
  Constant4/1 -> Mux1/3
  Relational/1 -> Mux1/1
  Constant3/1 -> Relational/1

== system rpoco16/ADC's/sat8 ==
  In2 : Inport
  Constant3 : xbsIndex_r4/Constant  const=-1  gui_display_data_type=Fixed-point  arith_type=Signed (2's comp)  n_bits=8  bin_pt=7  preci_type=Single  exp_width=8  frac_width=24  explicit_period=off  period=1  equ=P=C  opselect=C  inp2=PCIN>>17  opr=+  inp1=P  carry=CIN  dbl_ovrd=off  block_type=constant
      settings: block_version=11.4
  Constant4 : xbsIndex_r4/Constant  const=-127/128.  gui_display_data_type=Fixed-point  arith_type=Signed (2's comp)  n_bits=8  bin_pt=7  preci_type=Single  exp_width=8  frac_width=24  explicit_period=off  period=1  equ=P=C  opselect=C  inp2=PCIN>>17  opr=+  inp1=P  carry=CIN  dbl_ovrd=off  block_type=constant
      settings: block_version=11.4
  Mux1 : xbsIndex_r4/Mux  inputs=2  en=off  latency=0  precision=Full  arith_type=Unsigned  n_bits=16  bin_pt=14  quantization=Truncate  overflow=Wrap  dbl_ovrd=off  block_type=mux
      settings: block_version=11.4
  Relational : xbsIndex_r4/Relational  mode=a=b  en=off  latency=0  dbl_ovrd=off  block_type=relational
  Out1 : Outport
  wires:
  Constant3/1 -> Relational/1
  Relational/1 -> Mux1/1
  Constant4/1 -> Mux1/3
  Mux1/1 -> Out1/1
  In2/1 -> [d]
  [d] -> Relational/2
  [d] -> Mux1/2

== system rpoco16/ADC's/sat9 ==
  In2 : Inport
  Constant3 : xbsIndex_r4/Constant  const=-1  gui_display_data_type=Fixed-point  arith_type=Signed (2's comp)  n_bits=8  bin_pt=7  preci_type=Single  exp_width=8  frac_width=24  explicit_period=off  period=1  equ=P=C  opselect=C  inp2=PCIN>>17  opr=+  inp1=P  carry=CIN  dbl_ovrd=off  block_type=constant
      settings: block_version=11.4
  Constant4 : xbsIndex_r4/Constant  const=-127/128.  gui_display_data_type=Fixed-point  arith_type=Signed (2's comp)  n_bits=8  bin_pt=7  preci_type=Single  exp_width=8  frac_width=24  explicit_period=off  period=1  equ=P=C  opselect=C  inp2=PCIN>>17  opr=+  inp1=P  carry=CIN  dbl_ovrd=off  block_type=constant
      settings: block_version=11.4
  Mux1 : xbsIndex_r4/Mux  inputs=2  en=off  latency=0  precision=Full  arith_type=Unsigned  n_bits=16  bin_pt=14  quantization=Truncate  overflow=Wrap  dbl_ovrd=off  block_type=mux
      settings: block_version=11.4
  Relational : xbsIndex_r4/Relational  mode=a=b  en=off  latency=0  dbl_ovrd=off  block_type=relational
  Out1 : Outport
  wires:
  [d] -> Mux1/2
  [d] -> Relational/2
  In2/1 -> [d]
  Mux1/1 -> Out1/1
  Constant4/1 -> Mux1/3
  Relational/1 -> Mux1/1
  Constant3/1 -> Relational/1

== system rpoco16/Sync/arm ==
  sim_1 : Inport
  io_delay : xbsIndex_r4/Delay  rst=off  infoeditControl=Selection of Reset will increase slice count due to use of real FFs and instead of SRLs  en=off  latency=0  dbl_ovrd=off  reg_retiming=on  block_type=delay
  reint1 : xbsIndex_r4/Reinterpret  force_arith_type=on  arith_type=Unsigned  force_bin_pt=on  bin_pt=0  block_type=reinterpret
  rpoco16_Sync_arm_user_data_out : xbsIndex_r4/Gateway In  gui_display_data_type=Fixed-point  arith_type=Unsigned  n_bits=32  bin_pt=0  preci_type=Single  exp_width=8  frac_width=24  quantization="Round  (unbiased: +/- Inf)"  overflow=Saturate  period=1  dbl_ovrd=off  timing_constraint=None  locs_specified=off  LOCs={}  UseAsADC=off  ADCChannel='1'  inherit_from_input=off  hdl_port=on  block_type=gatewayin
  slice_reg : xbsIndex_r4/Slice  nbits=32  boolean_output=off  mode=Lower Bit Location + Width  bit1=0  base1=MSB of Input  bit0=0  base0=LSB of Input  dbl_ovrd=off  block_type=slice
  in_reg : Outport
  wires:
  rpoco16_Sync_arm_user_data_out/1 -> io_delay/1
  sim_1/1 -> rpoco16_Sync_arm_user_data_out/1
  io_delay/1 -> slice_reg/1
  slice_reg/1 -> reint1/1
  reint1/1 -> in_reg/1

== system rpoco16/Sync/posedge ==
  in : Inport
  Delay : xbsIndex_r4/Delay  rst=off  infoeditControl=Selection of Reset will increase slice count due to use of real FFs and instead of SRLs  en=off  latency=1  dbl_ovrd=off  reg_retiming=off  block_type=delay
      settings: xl_area=[0, 0, 0, 0, 0, 0, 0]
  Inverter : xbsIndex_r4/Inverter  en=off  latency=0  dbl_ovrd=off  block_type=inv
      settings: xl_area=[0, 0, 0, 0, 0, 0, 0]
  edge_op : xbsIndex_r4/Logical  logical_function=NOR  inputs=2  en=off  latency=0  precision=Full  arith_type=Unsigned  n_bits=8  bin_pt=2  align_bp=on  dbl_ovrd=off  block_type=logical
      settings: xl_area=[0, 0, 0, 0, 0, 0, 0]
  out : Outport
  wires:
  Inverter/1 -> edge_op/1
  edge_op/1 -> out/1
  in/1 -> Inverter/1, Delay/1
  Delay/1 -> edge_op/2

== system rpoco16/Sync/posedge1 ==
  in : Inport
  Delay : xbsIndex_r4/Delay  rst=off  infoeditControl=Selection of Reset will increase slice count due to use of real FFs and instead of SRLs  en=off  latency=1  dbl_ovrd=off  reg_retiming=off  block_type=delay
      settings: xl_area=[0, 0, 0, 0, 0, 0, 0]
  Inverter : xbsIndex_r4/Inverter  en=off  latency=0  dbl_ovrd=off  block_type=inv
      settings: xl_area=[0, 0, 0, 0, 0, 0, 0]
  edge_op : xbsIndex_r4/Logical  logical_function=NOR  inputs=2  en=off  latency=0  precision=Full  arith_type=Unsigned  n_bits=8  bin_pt=2  align_bp=on  dbl_ovrd=off  block_type=logical
      settings: xl_area=[0, 0, 0, 0, 0, 0, 0]
  out : Outport
  wires:
  Inverter/1 -> edge_op/1
  edge_op/1 -> out/1
  in/1 -> Inverter/1, Delay/1
  Delay/1 -> edge_op/2

== system rpoco16/Sync/sync_pulse ==
  sim_1 : Inport
  io_delay : xbsIndex_r4/Delay  rst=off  infoeditControl=Selection of Reset will increase slice count due to use of real FFs and instead of SRLs  en=off  latency=0  dbl_ovrd=off  reg_retiming=on  block_type=delay
  reint1 : xbsIndex_r4/Reinterpret  force_arith_type=on  arith_type=Unsigned  force_bin_pt=on  bin_pt=0  block_type=reinterpret
  rpoco16_Sync_sync_pulse_user_data_out : xbsIndex_r4/Gateway In  gui_display_data_type=Fixed-point  arith_type=Unsigned  n_bits=32  bin_pt=0  preci_type=Single  exp_width=8  frac_width=24  quantization="Round  (unbiased: +/- Inf)"  overflow=Saturate  period=1  dbl_ovrd=off  timing_constraint=None  locs_specified=off  LOCs={}  UseAsADC=off  ADCChannel='1'  inherit_from_input=off  hdl_port=on  block_type=gatewayin
  slice_reg : xbsIndex_r4/Slice  nbits=32  boolean_output=off  mode=Lower Bit Location + Width  bit1=0  base1=MSB of Input  bit0=0  base0=LSB of Input  dbl_ovrd=off  block_type=slice
  in_reg : Outport
  wires:
  rpoco16_Sync_sync_pulse_user_data_out/1 -> io_delay/1
  sim_1/1 -> rpoco16_Sync_sync_pulse_user_data_out/1
  io_delay/1 -> slice_reg/1
  slice_reg/1 -> reint1/1
  reint1/1 -> in_reg/1

== system rpoco16/Sync/sync_sel ==
  sim_1 : Inport
  io_delay : xbsIndex_r4/Delay  rst=off  infoeditControl=Selection of Reset will increase slice count due to use of real FFs and instead of SRLs  en=off  latency=0  dbl_ovrd=off  reg_retiming=on  block_type=delay
  reint1 : xbsIndex_r4/Reinterpret  force_arith_type=on  arith_type=Unsigned  force_bin_pt=on  bin_pt=0  block_type=reinterpret
  rpoco16_Sync_sync_sel_user_data_out : xbsIndex_r4/Gateway In  gui_display_data_type=Fixed-point  arith_type=Unsigned  n_bits=32  bin_pt=0  preci_type=Single  exp_width=8  frac_width=24  quantization="Round  (unbiased: +/- Inf)"  overflow=Saturate  period=1  dbl_ovrd=off  timing_constraint=None  locs_specified=off  LOCs={}  UseAsADC=off  ADCChannel='1'  inherit_from_input=off  hdl_port=on  block_type=gatewayin
  slice_reg : xbsIndex_r4/Slice  nbits=32  boolean_output=off  mode=Lower Bit Location + Width  bit1=0  base1=MSB of Input  bit0=0  base0=LSB of Input  dbl_ovrd=off  block_type=slice
  in_reg : Outport
  wires:
  rpoco16_Sync_sync_sel_user_data_out/1 -> io_delay/1
  sim_1/1 -> rpoco16_Sync_sync_sel_user_data_out/1
  io_delay/1 -> slice_reg/1
  slice_reg/1 -> reint1/1
  reint1/1 -> in_reg/1

== system rpoco16/WGNs/noise0 ==
  seed : Inport
  ld : Inport  Port=2
  Reinterpret : xbsIndex_r4/Reinterpret  force_arith_type=off  arith_type=Unsigned  force_bin_pt=on  bin_pt=7  block_type=reinterpret
      settings: infoedit="Changes signal type without altering the binary representation.   You can changed the signal between signed and unsigned, and relocate the binary point.<P><P>Hardware notes: In hardware this block costs nothing.<P><P>Example:  Suppose the input is 6 bits wide, signed, with 2 fractional bits, and the output is forced to unsigned with 0 fractional bits.  Then an input of -2.0 (1110.00 in binary 2's complement) becomes an output of 56 (111000 in binary)."  block_version=10.1.3
  Reinterpret1 : xbsIndex_r4/Reinterpret  force_arith_type=off  arith_type=Unsigned  force_bin_pt=on  bin_pt=7  block_type=reinterpret
      settings: infoedit="Changes signal type without altering the binary representation.   You can changed the signal between signed and unsigned, and relocate the binary point.<P><P>Hardware notes: In hardware this block costs nothing.<P><P>Example:  Suppose the input is 6 bits wide, signed, with 2 fractional bits, and the output is forced to unsigned with 0 fractional bits.  Then an input of -2.0 (1110.00 in binary 2's complement) becomes an output of 56 (111000 in binary)."  block_version=10.1.3
  Scale : xbsIndex_r4/Scale  scale_factor=4  dbl_ovrd=off  block_type=scale
      settings: infoedit=Scales input by a power of two by adjusting the binary point position.<P><P>Hardware notes: In hardware this block costs nothing.  block_version=10.1.3
  Scale1 : xbsIndex_r4/Scale  scale_factor=4  dbl_ovrd=off  block_type=scale
      settings: infoedit=Scales input by a power of two by adjusting the binary point position.<P><P>Hardware notes: In hardware this block costs nothing.  block_version=10.1.3
  convert : Subsystem  AncestorBlock=casper_library_misc/convert  mask(convert){bin_pt_in=10, n_bits_out=8, bin_pt_out=0, quantization=Round  (unbiased: +/- Inf), overflow=Wrap, latency=1}
      mask prompts: bin_pt_in "Binary Point In"; n_bits_out "Bit Width Out"; bin_pt_out "Binary Point Out"
      mask help:
      | Convert input value to the specified bit width and precision.
      |
      | Does not support upscaling number of fractional bits (eg 8_5 to 8_4 is ok, but not 8_4 to 8_5).
      mask init:
      | convert_init(gcb, ...
      |     'bin_pt_in',bin_pt_in, ...
      |     'n_bits_out',n_bits_out,...
      |     'bin_pt_out',bin_pt_out, ...
      |     'quantization',quantization,...
      |     'overflow',overflow,...
      |     'latency',latency);
      settings: AttributesFormatString=|
      | N_10 ==> 8_0
      | round inf, wrap
      | latency = 1
      mask Help:
      | <pre>
      | Description::
      | 
      | Outputs converted version of the input.
      | 
      | Mask Parameters::
      | 
      | Binary Point In (bin_pt_in): Specifies the binary point location in the input.
      | 
      | Bit Width Out (n_bits_out): Specifies the width of the output.
      | 
      | Binary Point Out (bin_pt_out): Specifies the binary point location in the output.
      | 
      | Quantization (quantization): Specifies quantization handling.
      | 
      | Overflow (overflow): Specifies overflow handling.
      | 
      | Latency (latency): Specifies the latency of the underlying adder block, which is the overall
      | latency of this block as well.
      | </pre>
      mask TypeOptions quantization: Truncate | Round  (unbiased: +/- Inf) | Round  (unbiased: Even Values) | Round  (unbiased: Zero) | Round  (unbiased: Odd Values) | Round  (biased: Up) | Round  (biased: Down)
      mask TypeOptions overflow: Wrap | Saturate | Error
  convert1 : Subsystem  AncestorBlock=casper_library_misc/convert  mask(convert){bin_pt_in=10, n_bits_out=8, bin_pt_out=0, quantization=Round  (unbiased: +/- Inf), overflow=Wrap, latency=1}
      mask prompts: bin_pt_in "Binary Point In"; n_bits_out "Bit Width Out"; bin_pt_out "Binary Point Out"
      mask help:
      | Convert input value to the specified bit width and precision.
      |
      | Does not support upscaling number of fractional bits (eg 8_5 to 8_4 is ok, but not 8_4 to 8_5).
      mask init: same as rpoco16/WGNs/noise0/convert
      settings: AttributesFormatString=|
      | N_10 ==> 8_0
      | round inf, wrap
      | latency = 1
      mask Help:
      | <pre>
      | Description::
      | 
      | Outputs converted version of the input.
      | 
      | Mask Parameters::
      | 
      | Binary Point In (bin_pt_in): Specifies the binary point location in the input.
      | 
      | Bit Width Out (n_bits_out): Specifies the width of the output.
      | 
      | Binary Point Out (bin_pt_out): Specifies the binary point location in the output.
      | 
      | Quantization (quantization): Specifies quantization handling.
      | 
      | Overflow (overflow): Specifies overflow handling.
      | 
      | Latency (latency): Specifies the latency of the underlying adder block, which is the overall
      | latency of this block as well.
      | </pre>
      mask TypeOptions quantization: Truncate | Round  (unbiased: +/- Inf) | Round  (unbiased: Even Values) | Round  (unbiased: Zero) | Round  (unbiased: Odd Values) | Round  (biased: Up) | Round  (biased: Down)
      mask TypeOptions overflow: Wrap | Saturate | Error
  wgn : casper_library_sources/White Gaussian Noise  seed=hex2dec('12345678')
  n1 : Outport
  n2 : Outport  Port=2
  wires:
  wgn/1 -> Scale/1
  wgn/2 -> Scale1/1
  convert/1(out) -> Reinterpret/1
  convert1/1(out) -> Reinterpret1/1
  seed/1 -> wgn/1
  ld/1 -> wgn/2
  Scale/1 -> convert/1(in)
  Scale1/1 -> convert1/1(in)
  Reinterpret/1 -> n1/1
  Reinterpret1/1 -> n2/1
